simulink model "PIDController_d3"  (R2022a)
settings: Solver=ode5  StartTime=0.0  StopTime=NaN  FixedStep=NaN  RelTol=1e-3
settings Model: Creator=Admin  LastModifiedBy=mquyet
settings SolverCC: AlgebraicLoopSolver=TrustRegion
settings DataIOCC: ReturnWorkspaceOutputs=off
settings DebuggingCC: UnconnectedInputMsg=warning  UnconnectedOutputMsg=warning  UnconnectedLineMsg=warning  SFMachineParentedDataDiag=warning  ArithmeticOperatorsInVariantConditions=warning
settings SFSimCC: SimUseLocalCustomCode=off  CustomCodeUndefinedFunction=UseInterfaceOnly
settings RTWCC: RTWUseLocalCustomCode=off
settings CodeAppCC: StateflowObjectComments=on

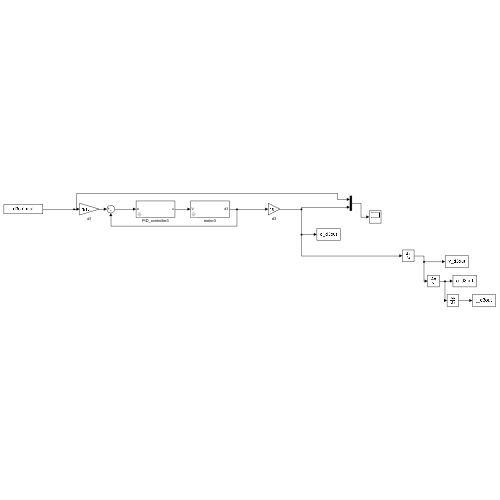
[thumbnail: Simulink's stored preview of the top-level diagram]
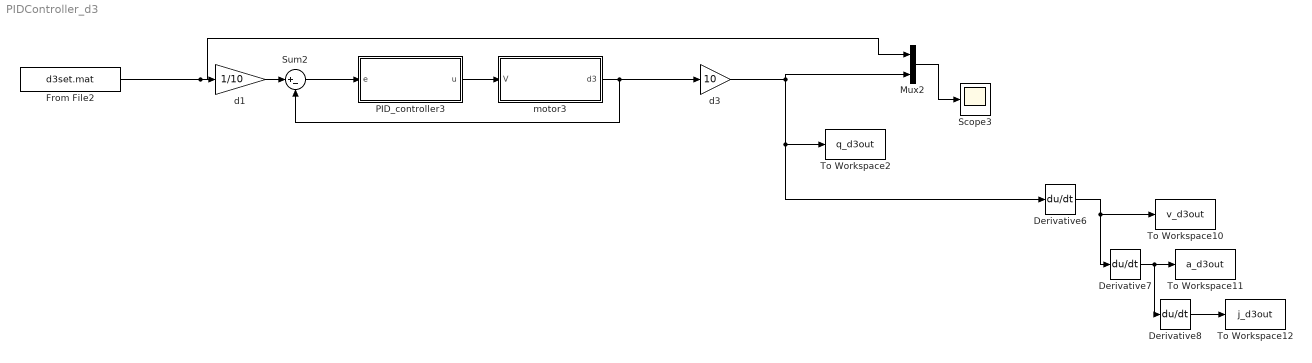
== system PIDController_d3 ==
  Derivative6 : Derivative
  Derivative7 : Derivative
  Derivative8 : Derivative
  From File2 : FromFile  FileName=d3set.mat
  Mux2 : Mux  Inputs=2
  PID_controller3 : Subsystem  mask{Kp=10000, Ki=0, Kd=100}
  Scope3 : Scope
  Sum2 : Sum  Inputs=|+-
  To Workspace10 : ToWorkspace  VariableName=v_d3out  SampleTime=-1
  To Workspace11 : ToWorkspace  VariableName=a_d3out  SampleTime=-1
  To Workspace12 : ToWorkspace  VariableName=j_d3out  SampleTime=-1
  To Workspace2 : ToWorkspace  VariableName=q_d3out  SampleTime=-1
  d1 : Gain  Gain=1/10
  d3 : Gain  Gain=10
  motor3 : Subsystem  mask{Ki=0.1, Kb=0.1, L=0.5, R=2, Jeff=0.02, Beff=0.2, N=100}
  wires:
  Sum2/1 -> PID_controller3/1(e)
  PID_controller3/1(u) -> motor3/1(V)
  From File2/1 -> Mux2/1, d1/1
  motor3/1(d3) -> d3/1, Sum2/2
  d3/1 -> Mux2/2, Derivative6/1, To Workspace2/1
  Derivative6/1 -> Derivative7/1, To Workspace10/1
  Derivative7/1 -> Derivative8/1, To Workspace11/1
  Derivative8/1 -> To Workspace12/1
  Mux2/1 -> Scope3/1
  d1/1 -> Sum2/1

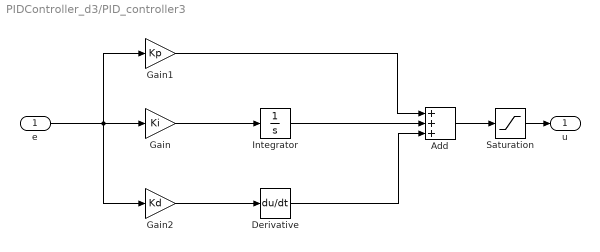
== system PIDController_d3/PID_controller3 ==
  e : Inport
  Add : Sum  Inputs=+++
  Derivative : Derivative
  Gain : Gain  Gain=Ki
  Gain1 : Gain  Gain=Kp
  Gain2 : Gain  Gain=Kd
  Integrator : Integrator
  Saturation : Saturate  UpperLimit=300  LowerLimit=-300
  u : Outport  VectorParamsAs1DForOutWhenUnconnected=off
  wires:
  e/1 -> Gain2/1, Gain1/1, Gain/1
  Gain/1 -> Integrator/1
  Gain2/1 -> Derivative/1
  Gain1/1 -> Add/1
  Integrator/1 -> Add/2
  Derivative/1 -> Add/3
  Add/1 -> Saturation/1
  Saturation/1 -> u/1

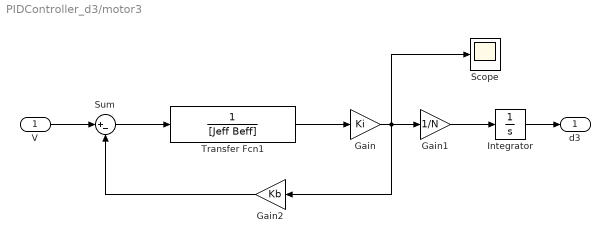
== system PIDController_d3/motor3 ==
  V : Inport
  Gain : Gain  Gain=Ki
  Gain1 : Gain  Gain=1/N
  Gain2 : Gain  Gain=Kb
  Integrator : Integrator
  Scope : Scope
  Sum : Sum  Inputs=|+-
  Transfer Fcn1 : TransferFcn  Denominator=[Jeff Beff]
  d3 : Outport  VectorParamsAs1DForOutWhenUnconnected=off
  wires:
  Transfer Fcn1/1 -> Gain/1
  Gain1/1 -> Integrator/1
  Integrator/1 -> d3/1
  Gain2/1 -> Sum/2
  V/1 -> Sum/1
  Sum/1 -> Transfer Fcn1/1
  Gain/1 -> Gain1/1, Gain2/1, Scope/1
